simulink model "slm1"  (R2018a)
settings: Solver=VariableStepAuto  StartTime=0.0  StopTime=10.0  RelTol=1e-9
values from neighbouring files (symbols this model uses):
  A = 0    [setup.m]
  b = 50    [setup.m]
  Kpe = 75    [setup.m]
  Kse = 135    [setup.m]
  M = [50,25,75]    [setup.m]
  z = [1,.5,5]    [setup.m]
undefined symbols (not defined in the file or in its folder): sigbuilder_block
settings Model: Creator=Pranav Maddula  LastModifiedBy=Pranav Maddula

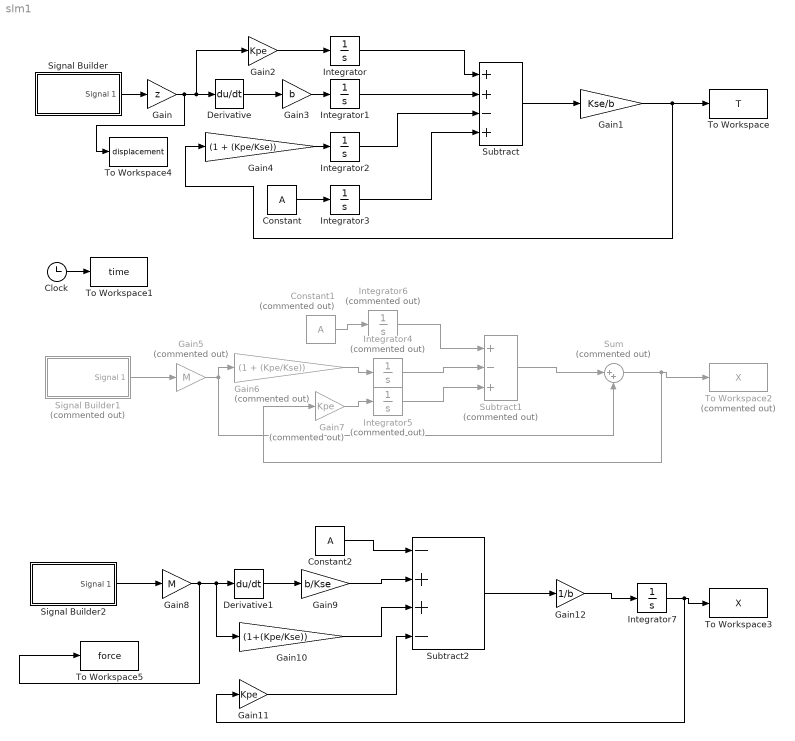
== system slm1 ==
  Clock : Clock
  Constant : Constant  Value=A
  Constant1 : Constant  Commented=on  Value=A
  Constant2 : Constant  Value=A
  Derivative : Derivative
  Derivative1 : Derivative
  Gain : Gain  Gain=z
  Gain1 : Gain  Gain=Kse/b
  Gain10 : Gain  Gain=(1+(Kpe/Kse))
  Gain11 : Gain  Gain=Kpe
  Gain12 : Gain  Gain=1/b
  Gain2 : Gain  Gain=Kpe
  Gain3 : Gain  Gain=b
  Gain4 : Gain  Gain=(1 + (Kpe/Kse))
  Gain5 : Gain  Commented=on  Gain=M
  Gain6 : Gain  Commented=on  Gain=(1 + (Kpe/Kse))
  Gain7 : Gain  Commented=on  Gain=Kpe
  Gain8 : Gain  Gain=M
  Gain9 : Gain  Gain=b/Kse
  Integrator{,1..3,7} (5 alike) : Integrator
  Integrator4 : Integrator  Commented=on
  Integrator5 : Integrator  Commented=on
  Integrator6 : Integrator  Commented=on
  Signal Builder : Subsystem  Tag=STV Subsys  LoadFcn=sigbuilder_block('load');  StartFcn=sigbuilder_block('start');  StopFcn=sigbuilder_block('stop');  ClipboardFcn=sigbuilder_block('clipboard');  mask(Sigbuilder block){tuvar=[0:10]}
      mask help: Simulink:masks:SigbuilderBlock_MD
      mask init:
      | if ~strcmp(get_param(bdroot(gcbh),'SimulationStatus'),'stopped') tuvar = sigbuilder_block('maskInit'); end
      settings: CopyFcn=sigbuilder_block('copy');  DeleteFcn=sigbuilder_block('delete');  ModelCloseFcn=sigbuilder_block('modelClose');  PreSaveFcn=sigbuilder_block('preSave');  PauseFcn=sigbuilder_block('pause');  ContinueFcn=sigbuilder_block('continue');  NameChangeFcn=sigbuilder_block('namechange');  OpenFcn=sigbuilder_block('open',[393.3 102.9 550.2 399.9 ]);  CloseFcn=sigbuilder_block('close');
      mask Display: plot(0, 0, 100, 100,[2, 2, 32, 32, 2], [68, 8, 8, 68, 68],[32, 2], [38, 38], [32, 19, 2],[53, 60, 44], [32, 17, 17, 2],[16, 16, 31, 31]);txt = getActiveGroup(gcbh);text(2, 100, txt,'verticalAlignment', 'top');
  Signal Builder1 : Subsystem  Tag=STV Subsys  Commented=on  LoadFcn=sigbuilder_block('load');  StartFcn=sigbuilder_block('start');  StopFcn=sigbuilder_block('stop');  ClipboardFcn=sigbuilder_block('clipboard');  mask(Sigbuilder block){tuvar=[0:10]}
      mask help: Simulink:masks:SigbuilderBlock_MD
      mask init:
      | if ~strcmp(get_param(bdroot(gcbh),'SimulationStatus'),'stopped') tuvar = sigbuilder_block('maskInit'); end
      settings: CopyFcn=sigbuilder_block('copy');  DeleteFcn=sigbuilder_block('delete');  ModelCloseFcn=sigbuilder_block('modelClose');  PreSaveFcn=sigbuilder_block('preSave');  PauseFcn=sigbuilder_block('pause');  ContinueFcn=sigbuilder_block('continue');  NameChangeFcn=sigbuilder_block('namechange');  OpenFcn=sigbuilder_block('open',[393.3 102.9 550.2 399.9 ]);  CloseFcn=sigbuilder_block('close');
      mask Display: plot(0, 0, 100, 100,[2, 2, 32, 32, 2], [68, 8, 8, 68, 68],[32, 2], [38, 38], [32, 19, 2],[53, 60, 44], [32, 17, 17, 2],[16, 16, 31, 31]);txt = getActiveGroup(gcbh);text(2, 100, txt,'verticalAlignment', 'top');
  Signal Builder2 : Subsystem  Tag=STV Subsys  LoadFcn=sigbuilder_block('load');  StartFcn=sigbuilder_block('start');  StopFcn=sigbuilder_block('stop');  ClipboardFcn=sigbuilder_block('clipboard');  mask(Sigbuilder block){tuvar=[0:10]}
      mask help: Simulink:masks:SigbuilderBlock_MD
      mask init:
      | if ~strcmp(get_param(bdroot(gcbh),'SimulationStatus'),'stopped') tuvar = sigbuilder_block('maskInit'); end
      settings: CopyFcn=sigbuilder_block('copy');  DeleteFcn=sigbuilder_block('delete');  ModelCloseFcn=sigbuilder_block('modelClose');  PreSaveFcn=sigbuilder_block('preSave');  PauseFcn=sigbuilder_block('pause');  ContinueFcn=sigbuilder_block('continue');  NameChangeFcn=sigbuilder_block('namechange');  OpenFcn=sigbuilder_block('open',[393.3 102.9 550.2 399.9 ]);  CloseFcn=sigbuilder_block('close');
      mask Display: plot(0, 0, 100, 100,[2, 2, 32, 32, 2], [68, 8, 8, 68, 68],[32, 2], [38, 38], [32, 19, 2],[53, 60, 44], [32, 17, 17, 2],[16, 16, 31, 31]);txt = getActiveGroup(gcbh);text(2, 100, txt,'verticalAlignment', 'top');
  Subtract : Sum  Inputs=++-+
  Subtract1 : Sum  Commented=on  Inputs=+-+
  Subtract2 : Sum  Inputs=-++-
  Sum : Sum  Commented=on  Inputs=|++
  To Workspace : ToWorkspace  VariableName=T  SampleTime=-1
  To Workspace1 : ToWorkspace  VariableName=time  SampleTime=-1
  To Workspace2 : ToWorkspace  Commented=on  VariableName=X  SampleTime=-1
  To Workspace3 : ToWorkspace  VariableName=X  SampleTime=-1
  To Workspace4 : ToWorkspace  VariableName=displacement  SampleTime=-1
  To Workspace5 : ToWorkspace  VariableName=force  SampleTime=-1
  wires:
  Signal Builder/1(Signal 1) -> Gain/1
  Subtract/1 -> Gain1/1
  Gain1/1 -> To Workspace/1, Gain4/1
  Gain/1 -> To Workspace4/1, Derivative/1, Gain2/1
  Gain4/1 -> Integrator2/1
  Integrator2/1 -> Subtract/3
  Constant/1 -> Integrator3/1
  Integrator3/1 -> Subtract/4
  Clock/1 -> To Workspace1/1
  Gain2/1 -> Integrator/1
  Integrator/1 -> Subtract/1
  Gain3/1 -> Integrator1/1
  Derivative/1 -> Gain3/1
  Integrator1/1 -> Subtract/2
  Signal Builder1/1(Signal 1) -> Gain5/1
  Gain6/1 -> Integrator4/1
  Subtract1/1 -> Sum/1
  Gain5/1 -> Sum/2, Gain6/1
  Integrator4/1 -> Subtract1/2
  Sum/1 -> Gain7/1, To Workspace2/1
  Gain7/1 -> Integrator5/1
  Integrator5/1 -> Subtract1/3
  Constant1/1 -> Integrator6/1
  Integrator6/1 -> Subtract1/1
  Signal Builder2/1(Signal 1) -> Gain8/1
  Gain8/1 -> To Workspace5/1, Gain10/1, Derivative1/1
  Derivative1/1 -> Gain9/1
  Gain9/1 -> Subtract2/2
  Constant2/1 -> Subtract2/1
  Gain10/1 -> Subtract2/3
  Gain11/1 -> Subtract2/4
  Gain12/1 -> Integrator7/1
  Integrator7/1 -> Gain11/1, To Workspace3/1
  Subtract2/1 -> Gain12/1

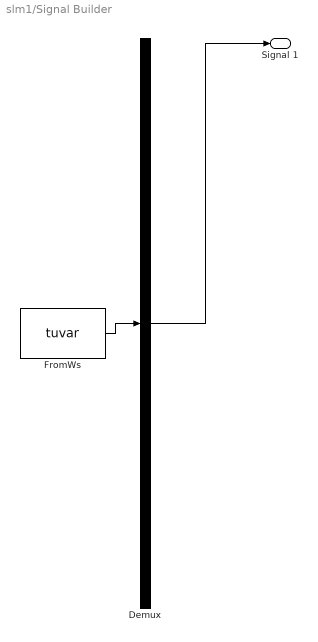
== system slm1/Signal Builder ==
  Demux : Demux  Tag=STV Demux  Outputs=1
  FromWs : FromWorkspace  Tag=STV FromWs  VariableName=tuvar  SampleTime=0
      SigBuilderData=|
      | common.afterFinalStr = 'Extrapolate'
      | common.sampleTime = 0
      | dataSet.timeRange = [0 10]
      | dataSet.name = 'Group 1'
      | sbobj.Groups.Name = 'Group 1'
      | sbobj.Groups.Signals.Name = 'Signal 1'
      | sbobj.Groups.Signals.XData = [0 0.05 3.05 3.1 6 10]
      | sbobj.Groups.Signals.YData = [0 1 1 0 0 0]
  Signal 1 : Outport  Tag=STV Outport
  wires:
  Demux/1 -> Signal 1/1
  FromWs/1 -> Demux/1

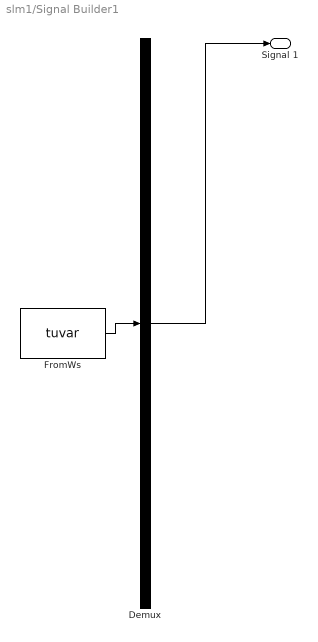
== system slm1/Signal Builder1 ==
  Demux : Demux  Tag=STV Demux  Outputs=1
  FromWs : FromWorkspace  Tag=STV FromWs  VariableName=tuvar  SampleTime=0
      SigBuilderData=|
      | common.afterFinalStr = 'Extrapolate'
      | common.sampleTime = 0
      | dataSet.timeRange = [0 10]
      | dataSet.name = 'Group 1'
      | sbobj.Groups.Name = 'Group 1'
      | sbobj.Groups.Signals.Name = 'Signal 1'
      | sbobj.Groups.Signals.XData = [0 0.05 3.05 3.1 6 10]
      | sbobj.Groups.Signals.YData = [0 1 1 0 0 0]
  Signal 1 : Outport  Tag=STV Outport
  wires:
  Demux/1 -> Signal 1/1
  FromWs/1 -> Demux/1

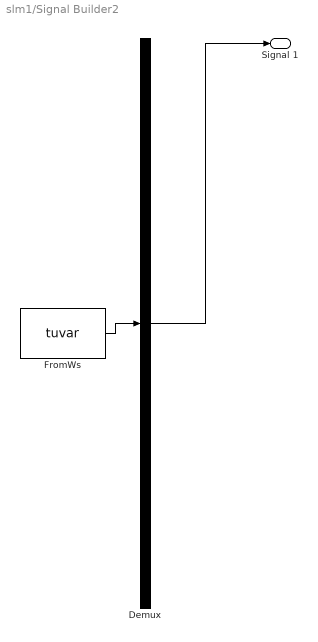
== system slm1/Signal Builder2 ==
  Demux : Demux  Tag=STV Demux  Outputs=1
  FromWs : FromWorkspace  Tag=STV FromWs  VariableName=tuvar  SampleTime=0
      SigBuilderData=|
      | common.afterFinalStr = 'Extrapolate'
      | common.sampleTime = 0
      | dataSet.timeRange = [0 10]
      | dataSet.name = 'Group 1'
      | sbobj.Groups.Name = 'Group 1'
      | sbobj.Groups.Signals.Name = 'Signal 1'
      | sbobj.Groups.Signals.XData = [0 0.05 3.05 3.1 6 10]
      | sbobj.Groups.Signals.YData = [0 1 1 0 0 0]
  Signal 1 : Outport  Tag=STV Outport
  wires:
  Demux/1 -> Signal 1/1
  FromWs/1 -> Demux/1
